simulink model "Referenced_Vehicle_Model"  (R2016b)
settings: Solver=ode3  StartTime=0.0  StopTime=1500  RelTol=1e-3
InitFcn:
  | % Call parameters initialization function
  | run optiTruck_init_sim.m;
StopFcn:
  | %optiTruck_post_sim;
  | %optiTruck_plot_sim;
undefined symbols (not defined in the file or in its folder): Cx, eff_final, eff_trans, f_0, gravity, K, mass, mass_effective, radius_wheel, rho, S, Ts, Velocity_initial
settings Model: Creator=engin  LastModifiedBy=engin.ozatay
settings DataIOCC: SaveFormat=StructureWithTime  SaveOutput=off  SaveTime=off
settings OptimizationCC: BlockReduction=off  BufferReuse=off  LifeSpan=inf
settings DebuggingCC: AlgebraicLoopMsg=none  UnconnectedInputMsg=none  UnconnectedOutputMsg=none  UnconnectedLineMsg=none  SFExecutionAtInitializationDiag=none
settings HardwareCC: ProdBitPerSizeT=32  ProdBitPerPtrDiffT=32  ProdWordSize=32  ProdHWDeviceType=Specified

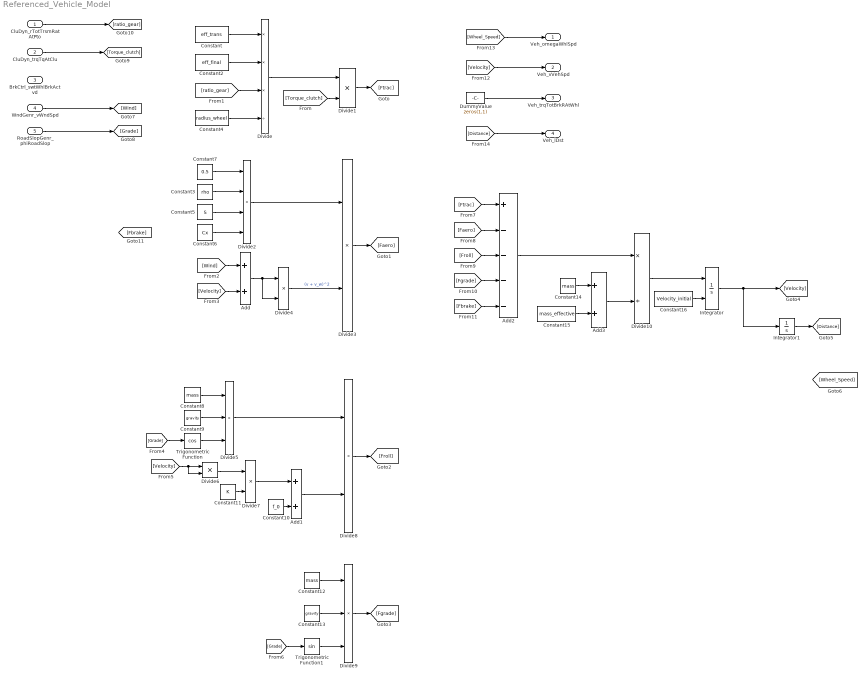
== system Referenced_Vehicle_Model ==
  CluDyn_rTotTrsmRatAtPto : Inport  OutDataTypeStr=double  PortDimensions=[1 1]  SampleTime=0
  CluDyn_trqTqAtClu : Inport  Port=2  OutDataTypeStr=double  PortDimensions=[1 1]  SampleTime=0
  BrkCtrl_swtWhlBrkActvd : Inport  Port=3  OutDataTypeStr=double  PortDimensions=1  SampleTime=0
  WndGenr_vWndSpd : Inport  Port=4  OutDataTypeStr=double  PortDimensions=[1 1]  SampleTime=0
  RoadSlopGenr_phiRoadSlop : Inport  Port=5  OutDataTypeStr=double  PortDimensions=[1 1]  SampleTime=0
  Add : Sum
  Add1 : Sum
  Add2 : Sum  Inputs=+----
  Add3 : Sum
  Constant : Constant  Value=eff_trans  SampleTime=Ts
  Constant10 : Constant  Value=f_0  SampleTime=Ts
  Constant11 : Constant  Value=K  SampleTime=Ts
  Constant12 : Constant  Value=mass  SampleTime=Ts
  Constant13 : Constant  Value=gravity  SampleTime=Ts
  Constant14 : Constant  Value=mass  SampleTime=Ts
  Constant15 : Constant  Value=mass_effective  SampleTime=Ts
  Constant16 : Constant  Value=Velocity_initial  SampleTime=Ts
  Constant2 : Constant  Value=eff_final  SampleTime=Ts
  Constant3 : Constant  Value=rho  SampleTime=Ts
  Constant4 : Constant  Value=radius_wheel  SampleTime=Ts
  Constant5 : Constant  Value=S  SampleTime=Ts
  Constant6 : Constant  Value=Cx  SampleTime=Ts
  Constant7 : Constant  Value=0.5  SampleTime=Ts
  Constant8 : Constant  Value=mass  SampleTime=Ts
  Constant9 : Constant  Value=gravity  SampleTime=Ts
  Divide : Product  Inputs=***/
  Divide{1,3..4,6..8} (6 alike) : Product  Inputs=**
  Divide10 : Product  Inputs=*/
  Divide2 : Product  Inputs=****
  Divide5 : Product  Inputs=***
  Divide9 : Product  Inputs=***
  DummyValue : Constant  Value=zeros(1,1)  VectorParams1D=off  OutDataTypeStr=double
  Integrator : Integrator  InitialConditionSource=external
  Integrator1 : Integrator
  Trigonometric Function : Trigonometry  Operator=cos
  Trigonometric Function1 : Trigonometry
  Veh_omegaWhlSpd : Outport  OutMin=0  OutMax=70  OutDataTypeStr=double  PortDimensions=1
  Veh_vVehSpd : Outport  Port=2  OutMin=0  OutMax=125  OutDataTypeStr=double  PortDimensions=[1 1]  SampleTime=0
  Veh_trqTotBrkRAtWhl : Outport  Port=3  OutMin=-32768  OutMax=32767  OutDataTypeStr=double  PortDimensions=[1 1]
  Veh_lDst : Outport  Port=4  OutMin=-2147483648  OutMax=2147483647  OutDataTypeStr=double  PortDimensions=[1 1]  SampleTime=0
  wires:
  [Velocity] -> Veh_vVehSpd/1
  [Wheel_Speed] -> Veh_omegaWhlSpd/1
  DummyValue/1 -> Veh_trqTotBrkRAtWhl/1
  WndGenr_vWndSpd/1 -> [Wind]
  RoadSlopGenr_phiRoadSlop/1 -> [Grade]
  Constant2/1 -> Divide/2
  [Torque_clutch] -> Divide1/2
  [ratio_gear] -> Divide/3
  Divide/1 -> Divide1/1
  Constant4/1 -> Divide/4
  Divide1/1 -> [Ftrac]
  Constant/1 -> Divide/1
  Add/1 -> Divide4/1, Divide4/2
  Divide3/1 -> [Faero]
  [Wind] -> Add/1
  Constant3/1 -> Divide2/2
  Constant5/1 -> Divide2/3
  Constant7/1 -> Divide2/1
  Divide2/1 -> Divide3/1
  [Velocity] -> Add/2
  Constant6/1 -> Divide2/4
  Divide4/1 -> Divide3/2  "(v + v_w)^2"
  Constant9/1 -> Divide5/2
  Add1/1 -> Divide8/2
  Divide7/1 -> Add1/1
  Constant8/1 -> Divide5/1
  Constant11/1 -> Divide7/2
  Divide6/1 -> Divide7/1
  Divide5/1 -> Divide8/1
  [Grade] -> Trigonometric Function/1
  Constant10/1 -> Add1/2
  Trigonometric Function/1 -> Divide5/3
  [Velocity] -> Divide6/1, Divide6/2
  Divide8/1 -> [Froll]
  Trigonometric Function1/1 -> Divide9/3
  Divide9/1 -> [Fgrade]
  Constant12/1 -> Divide9/1
  [Grade] -> Trigonometric Function1/1
  Constant13/1 -> Divide9/2
  Constant16/1 -> Integrator/2
  Divide10/1 -> Integrator/1
  [Froll] -> Add2/3
  Integrator/1 -> Integrator1/1, [Velocity]
  [Fbrake] -> Add2/5
  Add2/1 -> Divide10/1
  Constant15/1 -> Add3/2
  Constant14/1 -> Add3/1
  [Fgrade] -> Add2/4
  Add3/1 -> Divide10/2
  Integrator1/1 -> [Distance]
  [Faero] -> Add2/2
  [Ftrac] -> Add2/1
  CluDyn_trqTqAtClu/1 -> [Torque_clutch]
  CluDyn_rTotTrsmRatAtPto/1 -> [ratio_gear]
  [Distance] -> Veh_lDst/1
